simulink model "Gong_test"  (R2021b)
settings: Solver=VariableStepAuto  StartTime=0.0  StopTime=5  RelTol=1e-3
settings Model: Creator=rhdej  LastModifiedBy=rhdej

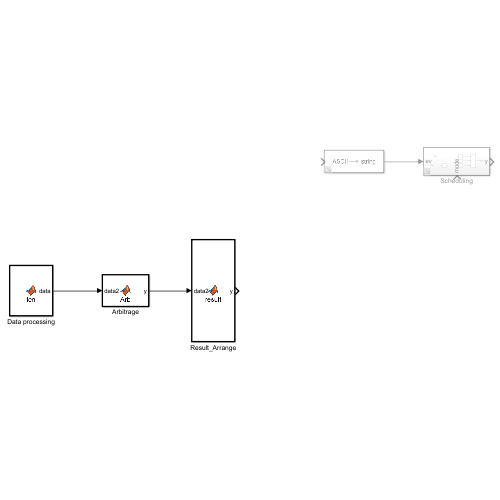
[thumbnail: Simulink's stored preview of the top-level diagram]
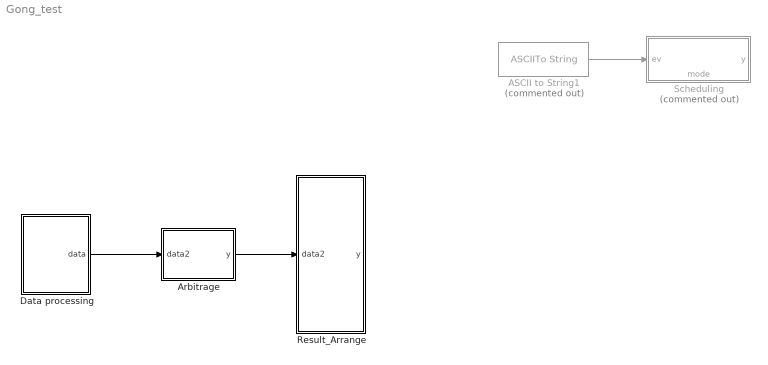
== system Gong_test ==
  ASCII to String1 : ASCIIToString  Commented=on
  Arbitrage : MATLAB Function  TreatAsAtomicUnit=on
  Data processing : MATLAB Function  TreatAsAtomicUnit=on
  Result_Arrange : MATLAB Function  TreatAsAtomicUnit=on
  Scheduling : Subsystem  Commented=on
      settings: PortSchema="{\"entries\":[{\"content\":{\"sides\":[{\"content\":{\"connectorIds\":[\"In1\"]},\"type\":\"ConnectorPlacement.EquallySpacedRectSide\",\"uuid\":\"d9aa8e7f-65ef-43bf-a654-7b3a6801d8a5\"},{\"content\":{\"connectorIds\":[\"Out1\"],\"side\":\"RIGHT\"},\"type\":\"ConnectorPlacement.EquallySpacedRectSide\",\"uuid\":\"e2073d63-3e33-4b33-bd20-152eb08a8602\"},{\"content\":{\"connectorIds\":[],\"side\":\"TOP\"},\"type\":\"ConnectorPlacement.EquallySpacedRectSide\",\"uuid\":\"055e1408-1ac8-4d97-be0b-843d7d62c121\"},{\"content\":{\"connectorIds\":[\"In2\"],\"side\":\"BOTTOM\"},\"type\":\"ConnectorPlacement.EquallySpacedRectSide\",\"uuid\":\"e2087943-3714-4c03-a00f-69d98931aa96\"}]},\"type\":\"ConnectorPlacement.EquallySpacedConnector\",\"uuid\":\"f1c97bcc-e04f-4d04-a5e3-5c4b657745ff\"}],\"packageUris\":[\"http://schema.mathworks.com/mf0/Connector/R2020b\"],\"version\":\"1.0\"}"
  wires:
  ASCII to String1/1 -> Scheduling/1(ev)
  Arbitrage/1(y) -> Result_Arrange/1(data2)
  Data processing/1(data) -> Arbitrage/1(data2)

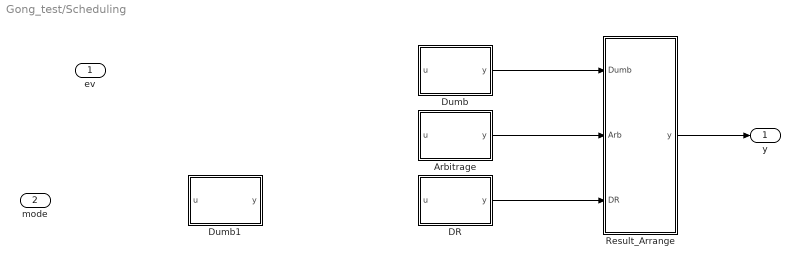
== system Gong_test/Scheduling ==
  ev : Inport
  mode : Inport  Port=2
  Arbitrage : MATLAB Function  TreatAsAtomicUnit=on
  DR : MATLAB Function  TreatAsAtomicUnit=on
  Dumb : MATLAB Function  TreatAsAtomicUnit=on
  Dumb1 : MATLAB Function  TreatAsAtomicUnit=on
  Result_Arrange : MATLAB Function  TreatAsAtomicUnit=on
  y : Outport
  wires:
  Result_Arrange/1(y) -> y/1
  Dumb/1(y) -> Result_Arrange/1(Dumb)
  Arbitrage/1(y) -> Result_Arrange/2(Arb)
  DR/1(y) -> Result_Arrange/3(DR)

== matlab function Gong_test/Scheduling/Arbitrage ==
  data: u input; y output
function y = Arb(u)
coder.extrinsic("readmatrix")
coder.extrinsic("intlinprog")

input = readmatrix(u);

== matlab function Gong_test/Data processing ==
  data: data output
function data = fcn
coder.extrinsic("readtable")
coder.extrinsic("readmatrix")
coder.extrinsic("writematrix")

input_ev = readmatrix("input/evConfig.csv");
mode = zeros(length(input_ev),1);
mode(:,1) = input_ev(:,13);

writematrix(input_ev,'tou.csv');
filename1 = 'ev.csv';
data = uint8(filename1);

== matlab function Gong_test/Scheduling/DR ==
  data: u input; y output
function y = DR(u)
coder.extrinsic("readmatrix")
coder.extrinsic("intlinprog")

input = readmatrix(u);

== matlab function Gong_test/Scheduling/Dumb ==
  data: u input; y output
function y = Dumb(u)
%Day : 1, ID : 2, Cap : 3, Init : 4, Target : 5, Min : 6, Max : 7, In : 8,
%Out : 9, Pmin : 10, Pmax : 11, Mode : 12, Massive option : 13
coder.extrinsic("readmatrix")
tou = readmatrix("input/tou.csv");


%Power 빈칸 만들기
power = zeros(length(ev));
%

input = readmatrix(u);

== matlab function Gong_test/Scheduling/Result_Arrange ==
  data: Dumb input; y output; Arb input; DR input
function y = fcn(Dumb, Arb, DR)
coder.extrinsic("readmatrix")
coder.extrinsic("intlinprog")

input = readmatrix(u);

== matlab function Gong_test/Scheduling/Dumb1 ==
  data: u input; y output
function y = Dumb(u)
coder.extrinsic("readmatrix")
coder.extrinsic("intlinprog")



input = readmatrix(u);

== matlab function Gong_test/Arbitrage ==
  data: y output; data2 input
function y = Arb(data2)
coder.extrinsic("readmatrix")
coder.extrinsic("intlinprog")

input = readmatrix(u);

== matlab function Gong_test/Result_Arrange ==
  data: y output; data2 input
function y = result(data2)
coder.extrinsic("readmatrix")
coder.extrinsic("intlinprog")

input = readmatrix(u);
